simulink model "c00009M_harness"  (R2018a)
settings: Solver=FixedStepAuto  StartTime=0.0  StopTime=300  FixedStep=0.1  RelTol=1e-3
undefined symbols (not defined in the file): A1, hmax, PriorityTank, R1, R2, sigbuilder_block
(part 3 of 29)

== system c00009M_harness/Eval226 ==
  In1 : Inport
  In2 : Inport  Port=2
  Constant3 : Constant
  Data Type Conversion : DataTypeConversion
  Data Type Conversion1 : DataTypeConversion
  Memory1 : Memory  InitialCondition=1
  Memory2 : Memory  InitialCondition=1
  MinMax : MinMax  Inputs=3
  MinMax1 : MinMax  Inputs=2
  MinMax2 : MinMax  Inputs=2
  ROOut1 : RelationalOperator  Operator===  OutDataTypeStr=boolean  RndMeth=Simplest
  ROOut2 : RelationalOperator  Operator===  OutDataTypeStr=boolean  RndMeth=Simplest
  Out1 : Outport
  wires:
  Data Type Conversion1/1 -> MinMax2/1
  Data Type Conversion/1 -> MinMax1/1
  MinMax1/1 -> Memory1/1, MinMax/1
  MinMax2/1 -> MinMax/2, Memory2/1
  ROOut1/1 -> Data Type Conversion/1
  Memory2/1 -> MinMax2/2
  ROOut2/1 -> Data Type Conversion1/1
  Memory1/1 -> MinMax1/2
  [out2] -> ROOut2/2
  In1/1 -> ROOut1/1
  In2/1 -> ROOut2/1
  [out1] -> ROOut1/2
  MinMax/1 -> Out1/1
  Constant3/1 -> MinMax/3

== system c00009M_harness/Eval227 ==
  In1 : Inport
  In2 : Inport  Port=2
  Constant3 : Constant
  Data Type Conversion : DataTypeConversion
  Data Type Conversion1 : DataTypeConversion
  Memory1 : Memory  InitialCondition=1
  Memory2 : Memory  InitialCondition=1
  MinMax : MinMax  Inputs=3
  MinMax1 : MinMax  Inputs=2
  MinMax2 : MinMax  Inputs=2
  ROOut1 : RelationalOperator  Operator===  OutDataTypeStr=boolean  RndMeth=Simplest
  ROOut2 : RelationalOperator  Operator===  OutDataTypeStr=boolean  RndMeth=Simplest
  Out1 : Outport
  wires:
  Data Type Conversion1/1 -> MinMax2/1
  Data Type Conversion/1 -> MinMax1/1
  MinMax1/1 -> Memory1/1, MinMax/1
  MinMax2/1 -> MinMax/2, Memory2/1
  ROOut1/1 -> Data Type Conversion/1
  Memory2/1 -> MinMax2/2
  ROOut2/1 -> Data Type Conversion1/1
  Memory1/1 -> MinMax1/2
  [out2] -> ROOut2/2
  In1/1 -> ROOut1/1
  In2/1 -> ROOut2/1
  [out1] -> ROOut1/2
  MinMax/1 -> Out1/1
  Constant3/1 -> MinMax/3

== system c00009M_harness/Eval228 ==
  In1 : Inport
  In2 : Inport  Port=2
  Constant3 : Constant
  Data Type Conversion : DataTypeConversion
  Data Type Conversion1 : DataTypeConversion
  Memory1 : Memory  InitialCondition=1
  Memory2 : Memory  InitialCondition=1
  MinMax : MinMax  Inputs=3
  MinMax1 : MinMax  Inputs=2
  MinMax2 : MinMax  Inputs=2
  ROOut1 : RelationalOperator  Operator===  OutDataTypeStr=boolean  RndMeth=Simplest
  ROOut2 : RelationalOperator  Operator===  OutDataTypeStr=boolean  RndMeth=Simplest
  Out1 : Outport
  wires:
  Data Type Conversion1/1 -> MinMax2/1
  Data Type Conversion/1 -> MinMax1/1
  MinMax1/1 -> Memory1/1, MinMax/1
  MinMax2/1 -> MinMax/2, Memory2/1
  ROOut1/1 -> Data Type Conversion/1
  Memory2/1 -> MinMax2/2
  ROOut2/1 -> Data Type Conversion1/1
  Memory1/1 -> MinMax1/2
  [out2] -> ROOut2/2
  In1/1 -> ROOut1/1
  In2/1 -> ROOut2/1
  [out1] -> ROOut1/2
  MinMax/1 -> Out1/1
  Constant3/1 -> MinMax/3

== system c00009M_harness/Eval229 ==
  In1 : Inport
  In2 : Inport  Port=2
  Constant3 : Constant
  Data Type Conversion : DataTypeConversion
  Data Type Conversion1 : DataTypeConversion
  Memory1 : Memory  InitialCondition=1
  Memory2 : Memory  InitialCondition=1
  MinMax : MinMax  Inputs=3
  MinMax1 : MinMax  Inputs=2
  MinMax2 : MinMax  Inputs=2
  ROOut1 : RelationalOperator  Operator===  OutDataTypeStr=boolean  RndMeth=Simplest
  ROOut2 : RelationalOperator  Operator===  OutDataTypeStr=boolean  RndMeth=Simplest
  Out1 : Outport
  wires:
  Data Type Conversion1/1 -> MinMax2/1
  Data Type Conversion/1 -> MinMax1/1
  MinMax1/1 -> Memory1/1, MinMax/1
  MinMax2/1 -> MinMax/2, Memory2/1
  ROOut1/1 -> Data Type Conversion/1
  Memory2/1 -> MinMax2/2
  ROOut2/1 -> Data Type Conversion1/1
  Memory1/1 -> MinMax1/2
  [out2] -> ROOut2/2
  In1/1 -> ROOut1/1
  In2/1 -> ROOut2/1
  [out1] -> ROOut1/2
  MinMax/1 -> Out1/1
  Constant3/1 -> MinMax/3

== system c00009M_harness/Eval45 ==
  In1 : Inport
  In2 : Inport  Port=2
  Constant3 : Constant
  Data Type Conversion : DataTypeConversion
  Data Type Conversion1 : DataTypeConversion
  Memory1 : Memory  InitialCondition=1
  Memory2 : Memory  InitialCondition=1
  MinMax : MinMax  Inputs=3
  MinMax1 : MinMax  Inputs=2
  MinMax2 : MinMax  Inputs=2
  ROOut1 : RelationalOperator  Operator===  OutDataTypeStr=boolean  RndMeth=Simplest
  ROOut2 : RelationalOperator  Operator===  OutDataTypeStr=boolean  RndMeth=Simplest
  Out1 : Outport
  wires:
  Data Type Conversion1/1 -> MinMax2/1
  Data Type Conversion/1 -> MinMax1/1
  MinMax1/1 -> Memory1/1, MinMax/1
  MinMax2/1 -> MinMax/2, Memory2/1
  ROOut1/1 -> Data Type Conversion/1
  Memory2/1 -> MinMax2/2
  ROOut2/1 -> Data Type Conversion1/1
  Memory1/1 -> MinMax1/2
  [out2] -> ROOut2/2
  In1/1 -> ROOut1/1
  In2/1 -> ROOut2/1
  [out1] -> ROOut1/2
  MinMax/1 -> Out1/1
  Constant3/1 -> MinMax/3

== system c00009M_harness/Eval46 ==
  In1 : Inport
  In2 : Inport  Port=2
  Constant3 : Constant
  Data Type Conversion : DataTypeConversion
  Data Type Conversion1 : DataTypeConversion
  Memory1 : Memory  InitialCondition=1
  Memory2 : Memory  InitialCondition=1
  MinMax : MinMax  Inputs=3
  MinMax1 : MinMax  Inputs=2
  MinMax2 : MinMax  Inputs=2
  ROOut1 : RelationalOperator  Operator===  OutDataTypeStr=boolean  RndMeth=Simplest
  ROOut2 : RelationalOperator  Operator===  OutDataTypeStr=boolean  RndMeth=Simplest
  Out1 : Outport
  wires:
  Data Type Conversion1/1 -> MinMax2/1
  Data Type Conversion/1 -> MinMax1/1
  MinMax1/1 -> Memory1/1, MinMax/1
  MinMax2/1 -> MinMax/2, Memory2/1
  ROOut1/1 -> Data Type Conversion/1
  Memory2/1 -> MinMax2/2
  ROOut2/1 -> Data Type Conversion1/1
  Memory1/1 -> MinMax1/2
  [out2] -> ROOut2/2
  In1/1 -> ROOut1/1
  In2/1 -> ROOut2/1
  [out1] -> ROOut1/2
  MinMax/1 -> Out1/1
  Constant3/1 -> MinMax/3

== system c00009M_harness/Eval47 ==
  In1 : Inport
  In2 : Inport  Port=2
  Constant3 : Constant
  Data Type Conversion : DataTypeConversion
  Data Type Conversion1 : DataTypeConversion
  Memory1 : Memory  InitialCondition=1
  Memory2 : Memory  InitialCondition=1
  MinMax : MinMax  Inputs=3
  MinMax1 : MinMax  Inputs=2
  MinMax2 : MinMax  Inputs=2
  ROOut1 : RelationalOperator  Operator===  OutDataTypeStr=boolean  RndMeth=Simplest
  ROOut2 : RelationalOperator  Operator===  OutDataTypeStr=boolean  RndMeth=Simplest
  Out1 : Outport
  wires:
  Data Type Conversion1/1 -> MinMax2/1
  Data Type Conversion/1 -> MinMax1/1
  MinMax1/1 -> Memory1/1, MinMax/1
  MinMax2/1 -> MinMax/2, Memory2/1
  ROOut1/1 -> Data Type Conversion/1
  Memory2/1 -> MinMax2/2
  ROOut2/1 -> Data Type Conversion1/1
  Memory1/1 -> MinMax1/2
  [out2] -> ROOut2/2
  In1/1 -> ROOut1/1
  In2/1 -> ROOut2/1
  [out1] -> ROOut1/2
  MinMax/1 -> Out1/1
  Constant3/1 -> MinMax/3

== system c00009M_harness/Eval48 ==
  In1 : Inport
  In2 : Inport  Port=2
  Constant3 : Constant
  Data Type Conversion : DataTypeConversion
  Data Type Conversion1 : DataTypeConversion
  Memory1 : Memory  InitialCondition=1
  Memory2 : Memory  InitialCondition=1
  MinMax : MinMax  Inputs=3
  MinMax1 : MinMax  Inputs=2
  MinMax2 : MinMax  Inputs=2
  ROOut1 : RelationalOperator  Operator===  OutDataTypeStr=boolean  RndMeth=Simplest
  ROOut2 : RelationalOperator  Operator===  OutDataTypeStr=boolean  RndMeth=Simplest
  Out1 : Outport
  wires:
  Data Type Conversion1/1 -> MinMax2/1
  Data Type Conversion/1 -> MinMax1/1
  MinMax1/1 -> Memory1/1, MinMax/1
  MinMax2/1 -> MinMax/2, Memory2/1
  ROOut1/1 -> Data Type Conversion/1
  Memory2/1 -> MinMax2/2
  ROOut2/1 -> Data Type Conversion1/1
  Memory1/1 -> MinMax1/2
  [out2] -> ROOut2/2
  In1/1 -> ROOut1/1
  In2/1 -> ROOut2/1
  [out1] -> ROOut1/2
  MinMax/1 -> Out1/1
  Constant3/1 -> MinMax/3

== system c00009M_harness/Eval49 ==
  In1 : Inport
  In2 : Inport  Port=2
  Constant3 : Constant
  Data Type Conversion : DataTypeConversion
  Data Type Conversion1 : DataTypeConversion
  Memory1 : Memory  InitialCondition=1
  Memory2 : Memory  InitialCondition=1
  MinMax : MinMax  Inputs=3
  MinMax1 : MinMax  Inputs=2
  MinMax2 : MinMax  Inputs=2
  ROOut1 : RelationalOperator  Operator===  OutDataTypeStr=boolean  RndMeth=Simplest
  ROOut2 : RelationalOperator  Operator===  OutDataTypeStr=boolean  RndMeth=Simplest
  Out1 : Outport
  wires:
  Data Type Conversion1/1 -> MinMax2/1
  Data Type Conversion/1 -> MinMax1/1
  MinMax1/1 -> Memory1/1, MinMax/1
  MinMax2/1 -> MinMax/2, Memory2/1
  ROOut1/1 -> Data Type Conversion/1
  Memory2/1 -> MinMax2/2
  ROOut2/1 -> Data Type Conversion1/1
  Memory1/1 -> MinMax1/2
  [out2] -> ROOut2/2
  In1/1 -> ROOut1/1
  In2/1 -> ROOut2/1
  [out1] -> ROOut1/2
  MinMax/1 -> Out1/1
  Constant3/1 -> MinMax/3

== system c00009M_harness/Eval50 ==
  In1 : Inport
  In2 : Inport  Port=2
  Constant3 : Constant
  Data Type Conversion : DataTypeConversion
  Data Type Conversion1 : DataTypeConversion
  Memory1 : Memory  InitialCondition=1
  Memory2 : Memory  InitialCondition=1
  MinMax : MinMax  Inputs=3
  MinMax1 : MinMax  Inputs=2
  MinMax2 : MinMax  Inputs=2
  ROOut1 : RelationalOperator  Operator===  OutDataTypeStr=boolean  RndMeth=Simplest
  ROOut2 : RelationalOperator  Operator===  OutDataTypeStr=boolean  RndMeth=Simplest
  Out1 : Outport
  wires:
  Data Type Conversion1/1 -> MinMax2/1
  Data Type Conversion/1 -> MinMax1/1
  MinMax1/1 -> Memory1/1, MinMax/1
  MinMax2/1 -> MinMax/2, Memory2/1
  ROOut1/1 -> Data Type Conversion/1
  Memory2/1 -> MinMax2/2
  ROOut2/1 -> Data Type Conversion1/1
  Memory1/1 -> MinMax1/2
  [out2] -> ROOut2/2
  In1/1 -> ROOut1/1
  In2/1 -> ROOut2/1
  [out1] -> ROOut1/2
  MinMax/1 -> Out1/1
  Constant3/1 -> MinMax/3

== system c00009M_harness/Eval51 ==
  In1 : Inport
  In2 : Inport  Port=2
  Constant3 : Constant
  Data Type Conversion : DataTypeConversion
  Data Type Conversion1 : DataTypeConversion
  Memory1 : Memory  InitialCondition=1
  Memory2 : Memory  InitialCondition=1
  MinMax : MinMax  Inputs=3
  MinMax1 : MinMax  Inputs=2
  MinMax2 : MinMax  Inputs=2
  ROOut1 : RelationalOperator  Operator===  OutDataTypeStr=boolean  RndMeth=Simplest
  ROOut2 : RelationalOperator  Operator===  OutDataTypeStr=boolean  RndMeth=Simplest
  Out1 : Outport
  wires:
  Data Type Conversion1/1 -> MinMax2/1
  Data Type Conversion/1 -> MinMax1/1
  MinMax1/1 -> Memory1/1, MinMax/1
  MinMax2/1 -> MinMax/2, Memory2/1
  ROOut1/1 -> Data Type Conversion/1
  Memory2/1 -> MinMax2/2
  ROOut2/1 -> Data Type Conversion1/1
  Memory1/1 -> MinMax1/2
  [out2] -> ROOut2/2
  In1/1 -> ROOut1/1
  In2/1 -> ROOut2/1
  [out1] -> ROOut1/2
  MinMax/1 -> Out1/1
  Constant3/1 -> MinMax/3

== system c00009M_harness/Eval52 ==
  In1 : Inport
  In2 : Inport  Port=2
  Constant3 : Constant
  Data Type Conversion : DataTypeConversion
  Data Type Conversion1 : DataTypeConversion
  Memory1 : Memory  InitialCondition=1
  Memory2 : Memory  InitialCondition=1
  MinMax : MinMax  Inputs=3
  MinMax1 : MinMax  Inputs=2
  MinMax2 : MinMax  Inputs=2
  ROOut1 : RelationalOperator  Operator===  OutDataTypeStr=boolean  RndMeth=Simplest
  ROOut2 : RelationalOperator  Operator===  OutDataTypeStr=boolean  RndMeth=Simplest
  Out1 : Outport
  wires:
  Data Type Conversion1/1 -> MinMax2/1
  Data Type Conversion/1 -> MinMax1/1
  MinMax1/1 -> Memory1/1, MinMax/1
  MinMax2/1 -> MinMax/2, Memory2/1
  ROOut1/1 -> Data Type Conversion/1
  Memory2/1 -> MinMax2/2
  ROOut2/1 -> Data Type Conversion1/1
  Memory1/1 -> MinMax1/2
  [out2] -> ROOut2/2
  In1/1 -> ROOut1/1
  In2/1 -> ROOut2/1
  [out1] -> ROOut1/2
  MinMax/1 -> Out1/1
  Constant3/1 -> MinMax/3

== system c00009M_harness/Eval53 ==
  In1 : Inport
  In2 : Inport  Port=2
  Constant3 : Constant
  Data Type Conversion : DataTypeConversion
  Data Type Conversion1 : DataTypeConversion
  Memory1 : Memory  InitialCondition=1
  Memory2 : Memory  InitialCondition=1
  MinMax : MinMax  Inputs=3
  MinMax1 : MinMax  Inputs=2
  MinMax2 : MinMax  Inputs=2
  ROOut1 : RelationalOperator  Operator===  OutDataTypeStr=boolean  RndMeth=Simplest
  ROOut2 : RelationalOperator  Operator===  OutDataTypeStr=boolean  RndMeth=Simplest
  Out1 : Outport
  wires:
  Data Type Conversion1/1 -> MinMax2/1
  Data Type Conversion/1 -> MinMax1/1
  MinMax1/1 -> Memory1/1, MinMax/1
  MinMax2/1 -> MinMax/2, Memory2/1
  ROOut1/1 -> Data Type Conversion/1
  Memory2/1 -> MinMax2/2
  ROOut2/1 -> Data Type Conversion1/1
  Memory1/1 -> MinMax1/2
  [out2] -> ROOut2/2
  In1/1 -> ROOut1/1
  In2/1 -> ROOut2/1
  [out1] -> ROOut1/2
  MinMax/1 -> Out1/1
  Constant3/1 -> MinMax/3

== system c00009M_harness/Eval54 ==
  In1 : Inport
  In2 : Inport  Port=2
  Constant3 : Constant
  Data Type Conversion : DataTypeConversion
  Data Type Conversion1 : DataTypeConversion
  Memory1 : Memory  InitialCondition=1
  Memory2 : Memory  InitialCondition=1
  MinMax : MinMax  Inputs=3
  MinMax1 : MinMax  Inputs=2
  MinMax2 : MinMax  Inputs=2
  ROOut1 : RelationalOperator  Operator===  OutDataTypeStr=boolean  RndMeth=Simplest
  ROOut2 : RelationalOperator  Operator===  OutDataTypeStr=boolean  RndMeth=Simplest
  Out1 : Outport
  wires:
  Data Type Conversion1/1 -> MinMax2/1
  Data Type Conversion/1 -> MinMax1/1
  MinMax1/1 -> Memory1/1, MinMax/1
  MinMax2/1 -> MinMax/2, Memory2/1
  ROOut1/1 -> Data Type Conversion/1
  Memory2/1 -> MinMax2/2
  ROOut2/1 -> Data Type Conversion1/1
  Memory1/1 -> MinMax1/2
  [out2] -> ROOut2/2
  In1/1 -> ROOut1/1
  In2/1 -> ROOut2/1
  [out1] -> ROOut1/2
  MinMax/1 -> Out1/1
  Constant3/1 -> MinMax/3

== system c00009M_harness/Eval55 ==
  In1 : Inport
  In2 : Inport  Port=2
  Constant3 : Constant
  Data Type Conversion : DataTypeConversion
  Data Type Conversion1 : DataTypeConversion
  Memory1 : Memory  InitialCondition=1
  Memory2 : Memory  InitialCondition=1
  MinMax : MinMax  Inputs=3
  MinMax1 : MinMax  Inputs=2
  MinMax2 : MinMax  Inputs=2
  ROOut1 : RelationalOperator  Operator===  OutDataTypeStr=boolean  RndMeth=Simplest
  ROOut2 : RelationalOperator  Operator===  OutDataTypeStr=boolean  RndMeth=Simplest
  Out1 : Outport
  wires:
  Data Type Conversion1/1 -> MinMax2/1
  Data Type Conversion/1 -> MinMax1/1
  MinMax1/1 -> Memory1/1, MinMax/1
  MinMax2/1 -> MinMax/2, Memory2/1
  ROOut1/1 -> Data Type Conversion/1
  Memory2/1 -> MinMax2/2
  ROOut2/1 -> Data Type Conversion1/1
  Memory1/1 -> MinMax1/2
  [out2] -> ROOut2/2
  In1/1 -> ROOut1/1
  In2/1 -> ROOut2/1
  [out1] -> ROOut1/2
  MinMax/1 -> Out1/1
  Constant3/1 -> MinMax/3

== system c00009M_harness/Eval57 ==
  In1 : Inport
  In2 : Inport  Port=2
  Constant3 : Constant
  Data Type Conversion : DataTypeConversion
  Data Type Conversion1 : DataTypeConversion
  Memory1 : Memory  InitialCondition=1
  Memory2 : Memory  InitialCondition=1
  MinMax : MinMax  Inputs=3
  MinMax1 : MinMax  Inputs=2
  MinMax2 : MinMax  Inputs=2
  ROOut1 : RelationalOperator  Operator===  OutDataTypeStr=boolean  RndMeth=Simplest
  ROOut2 : RelationalOperator  Operator===  OutDataTypeStr=boolean  RndMeth=Simplest
  Out1 : Outport
  wires:
  Data Type Conversion1/1 -> MinMax2/1
  Data Type Conversion/1 -> MinMax1/1
  MinMax1/1 -> Memory1/1, MinMax/1
  MinMax2/1 -> MinMax/2, Memory2/1
  ROOut1/1 -> Data Type Conversion/1
  Memory2/1 -> MinMax2/2
  ROOut2/1 -> Data Type Conversion1/1
  Memory1/1 -> MinMax1/2
  [out2] -> ROOut2/2
  In1/1 -> ROOut1/1
  In2/1 -> ROOut2/1
  [out1] -> ROOut1/2
  MinMax/1 -> Out1/1
  Constant3/1 -> MinMax/3

== system c00009M_harness/Eval58 ==
  In1 : Inport
  In2 : Inport  Port=2
  Constant3 : Constant
  Data Type Conversion : DataTypeConversion
  Data Type Conversion1 : DataTypeConversion
  Memory1 : Memory  InitialCondition=1
  Memory2 : Memory  InitialCondition=1
  MinMax : MinMax  Inputs=3
  MinMax1 : MinMax  Inputs=2
  MinMax2 : MinMax  Inputs=2
  ROOut1 : RelationalOperator  Operator===  OutDataTypeStr=boolean  RndMeth=Simplest
  ROOut2 : RelationalOperator  Operator===  OutDataTypeStr=boolean  RndMeth=Simplest
  Out1 : Outport
  wires:
  Data Type Conversion1/1 -> MinMax2/1
  Data Type Conversion/1 -> MinMax1/1
  MinMax1/1 -> Memory1/1, MinMax/1
  MinMax2/1 -> MinMax/2, Memory2/1
  ROOut1/1 -> Data Type Conversion/1
  Memory2/1 -> MinMax2/2
  ROOut2/1 -> Data Type Conversion1/1
  Memory1/1 -> MinMax1/2
  [out2] -> ROOut2/2
  In1/1 -> ROOut1/1
  In2/1 -> ROOut2/1
  [out1] -> ROOut1/2
  MinMax/1 -> Out1/1
  Constant3/1 -> MinMax/3

== system c00009M_harness/Eval59 ==
  In1 : Inport
  In2 : Inport  Port=2
  Constant3 : Constant
  Data Type Conversion : DataTypeConversion
  Data Type Conversion1 : DataTypeConversion
  Memory1 : Memory  InitialCondition=1
  Memory2 : Memory  InitialCondition=1
  MinMax : MinMax  Inputs=3
  MinMax1 : MinMax  Inputs=2
  MinMax2 : MinMax  Inputs=2
  ROOut1 : RelationalOperator  Operator===  OutDataTypeStr=boolean  RndMeth=Simplest
  ROOut2 : RelationalOperator  Operator===  OutDataTypeStr=boolean  RndMeth=Simplest
  Out1 : Outport
  wires:
  Data Type Conversion1/1 -> MinMax2/1
  Data Type Conversion/1 -> MinMax1/1
  MinMax1/1 -> Memory1/1, MinMax/1
  MinMax2/1 -> MinMax/2, Memory2/1
  ROOut1/1 -> Data Type Conversion/1
  Memory2/1 -> MinMax2/2
  ROOut2/1 -> Data Type Conversion1/1
  Memory1/1 -> MinMax1/2
  [out2] -> ROOut2/2
  In1/1 -> ROOut1/1
  In2/1 -> ROOut2/1
  [out1] -> ROOut1/2
  MinMax/1 -> Out1/1
  Constant3/1 -> MinMax/3

== system c00009M_harness/Eval60 ==
  In1 : Inport
  In2 : Inport  Port=2
  Constant3 : Constant
  Data Type Conversion : DataTypeConversion
  Data Type Conversion1 : DataTypeConversion
  Memory1 : Memory  InitialCondition=1
  Memory2 : Memory  InitialCondition=1
  MinMax : MinMax  Inputs=3
  MinMax1 : MinMax  Inputs=2
  MinMax2 : MinMax  Inputs=2
  ROOut1 : RelationalOperator  Operator===  OutDataTypeStr=boolean  RndMeth=Simplest
  ROOut2 : RelationalOperator  Operator===  OutDataTypeStr=boolean  RndMeth=Simplest
  Out1 : Outport
  wires:
  Data Type Conversion1/1 -> MinMax2/1
  Data Type Conversion/1 -> MinMax1/1
  MinMax1/1 -> Memory1/1, MinMax/1
  MinMax2/1 -> MinMax/2, Memory2/1
  ROOut1/1 -> Data Type Conversion/1
  Memory2/1 -> MinMax2/2
  ROOut2/1 -> Data Type Conversion1/1
  Memory1/1 -> MinMax1/2
  [out2] -> ROOut2/2
  In1/1 -> ROOut1/1
  In2/1 -> ROOut2/1
  [out1] -> ROOut1/2
  MinMax/1 -> Out1/1
  Constant3/1 -> MinMax/3

== system c00009M_harness/Eval61 ==
  In1 : Inport
  In2 : Inport  Port=2
  Constant3 : Constant
  Data Type Conversion : DataTypeConversion
  Data Type Conversion1 : DataTypeConversion
  Memory1 : Memory  InitialCondition=1
  Memory2 : Memory  InitialCondition=1
  MinMax : MinMax  Inputs=3
  MinMax1 : MinMax  Inputs=2
  MinMax2 : MinMax  Inputs=2
  ROOut1 : RelationalOperator  Operator===  OutDataTypeStr=boolean  RndMeth=Simplest
  ROOut2 : RelationalOperator  Operator===  OutDataTypeStr=boolean  RndMeth=Simplest
  Out1 : Outport
  wires:
  Data Type Conversion1/1 -> MinMax2/1
  Data Type Conversion/1 -> MinMax1/1
  MinMax1/1 -> Memory1/1, MinMax/1
  MinMax2/1 -> MinMax/2, Memory2/1
  ROOut1/1 -> Data Type Conversion/1
  Memory2/1 -> MinMax2/2
  ROOut2/1 -> Data Type Conversion1/1
  Memory1/1 -> MinMax1/2
  [out2] -> ROOut2/2
  In1/1 -> ROOut1/1
  In2/1 -> ROOut2/1
  [out1] -> ROOut1/2
  MinMax/1 -> Out1/1
  Constant3/1 -> MinMax/3

== system c00009M_harness/Eval62 ==
  In1 : Inport
  In2 : Inport  Port=2
  Constant3 : Constant
  Data Type Conversion : DataTypeConversion
  Data Type Conversion1 : DataTypeConversion
  Memory1 : Memory  InitialCondition=1
  Memory2 : Memory  InitialCondition=1
  MinMax : MinMax  Inputs=3
  MinMax1 : MinMax  Inputs=2
  MinMax2 : MinMax  Inputs=2
  ROOut1 : RelationalOperator  Operator===  OutDataTypeStr=boolean  RndMeth=Simplest
  ROOut2 : RelationalOperator  Operator===  OutDataTypeStr=boolean  RndMeth=Simplest
  Out1 : Outport
  wires:
  Data Type Conversion1/1 -> MinMax2/1
  Data Type Conversion/1 -> MinMax1/1
  MinMax1/1 -> Memory1/1, MinMax/1
  MinMax2/1 -> MinMax/2, Memory2/1
  ROOut1/1 -> Data Type Conversion/1
  Memory2/1 -> MinMax2/2
  ROOut2/1 -> Data Type Conversion1/1
  Memory1/1 -> MinMax1/2
  [out2] -> ROOut2/2
  In1/1 -> ROOut1/1
  In2/1 -> ROOut2/1
  [out1] -> ROOut1/2
  MinMax/1 -> Out1/1
  Constant3/1 -> MinMax/3

== system c00009M_harness/Eval63 ==
  In1 : Inport
  In2 : Inport  Port=2
  Constant3 : Constant
  Data Type Conversion : DataTypeConversion
  Data Type Conversion1 : DataTypeConversion
  Memory1 : Memory  InitialCondition=1
  Memory2 : Memory  InitialCondition=1
  MinMax : MinMax  Inputs=3
  MinMax1 : MinMax  Inputs=2
  MinMax2 : MinMax  Inputs=2
  ROOut1 : RelationalOperator  Operator===  OutDataTypeStr=boolean  RndMeth=Simplest
  ROOut2 : RelationalOperator  Operator===  OutDataTypeStr=boolean  RndMeth=Simplest
  Out1 : Outport
  wires:
  Data Type Conversion1/1 -> MinMax2/1
  Data Type Conversion/1 -> MinMax1/1
  MinMax1/1 -> Memory1/1, MinMax/1
  MinMax2/1 -> MinMax/2, Memory2/1
  ROOut1/1 -> Data Type Conversion/1
  Memory2/1 -> MinMax2/2
  ROOut2/1 -> Data Type Conversion1/1
  Memory1/1 -> MinMax1/2
  [out2] -> ROOut2/2
  In1/1 -> ROOut1/1
  In2/1 -> ROOut2/1
  [out1] -> ROOut1/2
  MinMax/1 -> Out1/1
  Constant3/1 -> MinMax/3

== system c00009M_harness/Eval64 ==
  In1 : Inport
  In2 : Inport  Port=2
  Constant3 : Constant
  Data Type Conversion : DataTypeConversion
  Data Type Conversion1 : DataTypeConversion
  Memory1 : Memory  InitialCondition=1
  Memory2 : Memory  InitialCondition=1
  MinMax : MinMax  Inputs=3
  MinMax1 : MinMax  Inputs=2
  MinMax2 : MinMax  Inputs=2
  ROOut1 : RelationalOperator  Operator===  OutDataTypeStr=boolean  RndMeth=Simplest
  ROOut2 : RelationalOperator  Operator===  OutDataTypeStr=boolean  RndMeth=Simplest
  Out1 : Outport
  wires:
  Data Type Conversion1/1 -> MinMax2/1
  Data Type Conversion/1 -> MinMax1/1
  MinMax1/1 -> Memory1/1, MinMax/1
  MinMax2/1 -> MinMax/2, Memory2/1
  ROOut1/1 -> Data Type Conversion/1
  Memory2/1 -> MinMax2/2
  ROOut2/1 -> Data Type Conversion1/1
  Memory1/1 -> MinMax1/2
  [out2] -> ROOut2/2
  In1/1 -> ROOut1/1
  In2/1 -> ROOut2/1
  [out1] -> ROOut1/2
  MinMax/1 -> Out1/1
  Constant3/1 -> MinMax/3

== system c00009M_harness/Eval65 ==
  In1 : Inport
  In2 : Inport  Port=2
  Constant3 : Constant
  Data Type Conversion : DataTypeConversion
  Data Type Conversion1 : DataTypeConversion
  Memory1 : Memory  InitialCondition=1
  Memory2 : Memory  InitialCondition=1
  MinMax : MinMax  Inputs=3
  MinMax1 : MinMax  Inputs=2
  MinMax2 : MinMax  Inputs=2
  ROOut1 : RelationalOperator  Operator===  OutDataTypeStr=boolean  RndMeth=Simplest
  ROOut2 : RelationalOperator  Operator===  OutDataTypeStr=boolean  RndMeth=Simplest
  Out1 : Outport
  wires:
  Data Type Conversion1/1 -> MinMax2/1
  Data Type Conversion/1 -> MinMax1/1
  MinMax1/1 -> Memory1/1, MinMax/1
  MinMax2/1 -> MinMax/2, Memory2/1
  ROOut1/1 -> Data Type Conversion/1
  Memory2/1 -> MinMax2/2
  ROOut2/1 -> Data Type Conversion1/1
  Memory1/1 -> MinMax1/2
  [out2] -> ROOut2/2
  In1/1 -> ROOut1/1
  In2/1 -> ROOut2/1
  [out1] -> ROOut1/2
  MinMax/1 -> Out1/1
  Constant3/1 -> MinMax/3

== system c00009M_harness/Eval66 ==
  In1 : Inport
  In2 : Inport  Port=2
  Constant3 : Constant
  Data Type Conversion : DataTypeConversion
  Data Type Conversion1 : DataTypeConversion
  Memory1 : Memory  InitialCondition=1
  Memory2 : Memory  InitialCondition=1
  MinMax : MinMax  Inputs=3
  MinMax1 : MinMax  Inputs=2
  MinMax2 : MinMax  Inputs=2
  ROOut1 : RelationalOperator  Operator===  OutDataTypeStr=boolean  RndMeth=Simplest
  ROOut2 : RelationalOperator  Operator===  OutDataTypeStr=boolean  RndMeth=Simplest
  Out1 : Outport
  wires:
  Data Type Conversion1/1 -> MinMax2/1
  Data Type Conversion/1 -> MinMax1/1
  MinMax1/1 -> Memory1/1, MinMax/1
  MinMax2/1 -> MinMax/2, Memory2/1
  ROOut1/1 -> Data Type Conversion/1
  Memory2/1 -> MinMax2/2
  ROOut2/1 -> Data Type Conversion1/1
  Memory1/1 -> MinMax1/2
  [out2] -> ROOut2/2
  In1/1 -> ROOut1/1
  In2/1 -> ROOut2/1
  [out1] -> ROOut1/2
  MinMax/1 -> Out1/1
  Constant3/1 -> MinMax/3

== system c00009M_harness/Eval67 ==
  In1 : Inport
  In2 : Inport  Port=2
  Constant3 : Constant
  Data Type Conversion : DataTypeConversion
  Data Type Conversion1 : DataTypeConversion
  Memory1 : Memory  InitialCondition=1
  Memory2 : Memory  InitialCondition=1
  MinMax : MinMax  Inputs=3
  MinMax1 : MinMax  Inputs=2
  MinMax2 : MinMax  Inputs=2
  ROOut1 : RelationalOperator  Operator===  OutDataTypeStr=boolean  RndMeth=Simplest
  ROOut2 : RelationalOperator  Operator===  OutDataTypeStr=boolean  RndMeth=Simplest
  Out1 : Outport
  wires:
  Data Type Conversion1/1 -> MinMax2/1
  Data Type Conversion/1 -> MinMax1/1
  MinMax1/1 -> Memory1/1, MinMax/1
  MinMax2/1 -> MinMax/2, Memory2/1
  ROOut1/1 -> Data Type Conversion/1
  Memory2/1 -> MinMax2/2
  ROOut2/1 -> Data Type Conversion1/1
  Memory1/1 -> MinMax1/2
  [out2] -> ROOut2/2
  In1/1 -> ROOut1/1
  In2/1 -> ROOut2/1
  [out1] -> ROOut1/2
  MinMax/1 -> Out1/1
  Constant3/1 -> MinMax/3

== system c00009M_harness/Eval68 ==
  In1 : Inport
  In2 : Inport  Port=2
  Constant3 : Constant
  Data Type Conversion : DataTypeConversion
  Data Type Conversion1 : DataTypeConversion
  Memory1 : Memory  InitialCondition=1
  Memory2 : Memory  InitialCondition=1
  MinMax : MinMax  Inputs=3
  MinMax1 : MinMax  Inputs=2
  MinMax2 : MinMax  Inputs=2
  ROOut1 : RelationalOperator  Operator===  OutDataTypeStr=boolean  RndMeth=Simplest
  ROOut2 : RelationalOperator  Operator===  OutDataTypeStr=boolean  RndMeth=Simplest
  Out1 : Outport
  wires:
  Data Type Conversion1/1 -> MinMax2/1
  Data Type Conversion/1 -> MinMax1/1
  MinMax1/1 -> Memory1/1, MinMax/1
  MinMax2/1 -> MinMax/2, Memory2/1
  ROOut1/1 -> Data Type Conversion/1
  Memory2/1 -> MinMax2/2
  ROOut2/1 -> Data Type Conversion1/1
  Memory1/1 -> MinMax1/2
  [out2] -> ROOut2/2
  In1/1 -> ROOut1/1
  In2/1 -> ROOut2/1
  [out1] -> ROOut1/2
  MinMax/1 -> Out1/1
  Constant3/1 -> MinMax/3

== system c00009M_harness/Eval69 ==
  In1 : Inport
  In2 : Inport  Port=2
  Constant3 : Constant
  Data Type Conversion : DataTypeConversion
  Data Type Conversion1 : DataTypeConversion
  Memory1 : Memory  InitialCondition=1
  Memory2 : Memory  InitialCondition=1
  MinMax : MinMax  Inputs=3
  MinMax1 : MinMax  Inputs=2
  MinMax2 : MinMax  Inputs=2
  ROOut1 : RelationalOperator  Operator===  OutDataTypeStr=boolean  RndMeth=Simplest
  ROOut2 : RelationalOperator  Operator===  OutDataTypeStr=boolean  RndMeth=Simplest
  Out1 : Outport
  wires:
  Data Type Conversion1/1 -> MinMax2/1
  Data Type Conversion/1 -> MinMax1/1
  MinMax1/1 -> Memory1/1, MinMax/1
  MinMax2/1 -> MinMax/2, Memory2/1
  ROOut1/1 -> Data Type Conversion/1
  Memory2/1 -> MinMax2/2
  ROOut2/1 -> Data Type Conversion1/1
  Memory1/1 -> MinMax1/2
  [out2] -> ROOut2/2
  In1/1 -> ROOut1/1
  In2/1 -> ROOut2/1
  [out1] -> ROOut1/2
  MinMax/1 -> Out1/1
  Constant3/1 -> MinMax/3

== system c00009M_harness/Eval70 ==
  In1 : Inport
  In2 : Inport  Port=2
  Constant3 : Constant
  Data Type Conversion : DataTypeConversion
  Data Type Conversion1 : DataTypeConversion
  Memory1 : Memory  InitialCondition=1
  Memory2 : Memory  InitialCondition=1
  MinMax : MinMax  Inputs=3
  MinMax1 : MinMax  Inputs=2
  MinMax2 : MinMax  Inputs=2
  ROOut1 : RelationalOperator  Operator===  OutDataTypeStr=boolean  RndMeth=Simplest
  ROOut2 : RelationalOperator  Operator===  OutDataTypeStr=boolean  RndMeth=Simplest
  Out1 : Outport
  wires:
  Data Type Conversion1/1 -> MinMax2/1
  Data Type Conversion/1 -> MinMax1/1
  MinMax1/1 -> Memory1/1, MinMax/1
  MinMax2/1 -> MinMax/2, Memory2/1
  ROOut1/1 -> Data Type Conversion/1
  Memory2/1 -> MinMax2/2
  ROOut2/1 -> Data Type Conversion1/1
  Memory1/1 -> MinMax1/2
  [out2] -> ROOut2/2
  In1/1 -> ROOut1/1
  In2/1 -> ROOut2/1
  [out1] -> ROOut1/2
  MinMax/1 -> Out1/1
  Constant3/1 -> MinMax/3

== system c00009M_harness/Eval71 ==
  In1 : Inport
  In2 : Inport  Port=2
  Constant3 : Constant
  Data Type Conversion : DataTypeConversion
  Data Type Conversion1 : DataTypeConversion
  Memory1 : Memory  InitialCondition=1
  Memory2 : Memory  InitialCondition=1
  MinMax : MinMax  Inputs=3
  MinMax1 : MinMax  Inputs=2
  MinMax2 : MinMax  Inputs=2
  ROOut1 : RelationalOperator  Operator===  OutDataTypeStr=boolean  RndMeth=Simplest
  ROOut2 : RelationalOperator  Operator===  OutDataTypeStr=boolean  RndMeth=Simplest
  Out1 : Outport
  wires:
  Data Type Conversion1/1 -> MinMax2/1
  Data Type Conversion/1 -> MinMax1/1
  MinMax1/1 -> Memory1/1, MinMax/1
  MinMax2/1 -> MinMax/2, Memory2/1
  ROOut1/1 -> Data Type Conversion/1
  Memory2/1 -> MinMax2/2
  ROOut2/1 -> Data Type Conversion1/1
  Memory1/1 -> MinMax1/2
  [out2] -> ROOut2/2
  In1/1 -> ROOut1/1
  In2/1 -> ROOut2/1
  [out1] -> ROOut1/2
  MinMax/1 -> Out1/1
  Constant3/1 -> MinMax/3

== system c00009M_harness/Eval72 ==
  In1 : Inport
  In2 : Inport  Port=2
  Constant3 : Constant
  Data Type Conversion : DataTypeConversion
  Data Type Conversion1 : DataTypeConversion
  Memory1 : Memory  InitialCondition=1
  Memory2 : Memory  InitialCondition=1
  MinMax : MinMax  Inputs=3
  MinMax1 : MinMax  Inputs=2
  MinMax2 : MinMax  Inputs=2
  ROOut1 : RelationalOperator  Operator===  OutDataTypeStr=boolean  RndMeth=Simplest
  ROOut2 : RelationalOperator  Operator===  OutDataTypeStr=boolean  RndMeth=Simplest
  Out1 : Outport
  wires:
  Data Type Conversion1/1 -> MinMax2/1
  Data Type Conversion/1 -> MinMax1/1
  MinMax1/1 -> Memory1/1, MinMax/1
  MinMax2/1 -> MinMax/2, Memory2/1
  ROOut1/1 -> Data Type Conversion/1
  Memory2/1 -> MinMax2/2
  ROOut2/1 -> Data Type Conversion1/1
  Memory1/1 -> MinMax1/2
  [out2] -> ROOut2/2
  In1/1 -> ROOut1/1
  In2/1 -> ROOut2/1
  [out1] -> ROOut1/2
  MinMax/1 -> Out1/1
  Constant3/1 -> MinMax/3

== system c00009M_harness/Eval73 ==
  In1 : Inport
  In2 : Inport  Port=2
  Constant3 : Constant
  Data Type Conversion : DataTypeConversion
  Data Type Conversion1 : DataTypeConversion
  Memory1 : Memory  InitialCondition=1
  Memory2 : Memory  InitialCondition=1
  MinMax : MinMax  Inputs=3
  MinMax1 : MinMax  Inputs=2
  MinMax2 : MinMax  Inputs=2
  ROOut1 : RelationalOperator  Operator===  OutDataTypeStr=boolean  RndMeth=Simplest
  ROOut2 : RelationalOperator  Operator===  OutDataTypeStr=boolean  RndMeth=Simplest
  Out1 : Outport
  wires:
  Data Type Conversion1/1 -> MinMax2/1
  Data Type Conversion/1 -> MinMax1/1
  MinMax1/1 -> Memory1/1, MinMax/1
  MinMax2/1 -> MinMax/2, Memory2/1
  ROOut1/1 -> Data Type Conversion/1
  Memory2/1 -> MinMax2/2
  ROOut2/1 -> Data Type Conversion1/1
  Memory1/1 -> MinMax1/2
  [out2] -> ROOut2/2
  In1/1 -> ROOut1/1
  In2/1 -> ROOut2/1
  [out1] -> ROOut1/2
  MinMax/1 -> Out1/1
  Constant3/1 -> MinMax/3

== system c00009M_harness/Eval74 ==
  In1 : Inport
  In2 : Inport  Port=2
  Constant3 : Constant
  Data Type Conversion : DataTypeConversion
  Data Type Conversion1 : DataTypeConversion
  Memory1 : Memory  InitialCondition=1
  Memory2 : Memory  InitialCondition=1
  MinMax : MinMax  Inputs=3
  MinMax1 : MinMax  Inputs=2
  MinMax2 : MinMax  Inputs=2
  ROOut1 : RelationalOperator  Operator===  OutDataTypeStr=boolean  RndMeth=Simplest
  ROOut2 : RelationalOperator  Operator===  OutDataTypeStr=boolean  RndMeth=Simplest
  Out1 : Outport
  wires:
  Data Type Conversion1/1 -> MinMax2/1
  Data Type Conversion/1 -> MinMax1/1
  MinMax1/1 -> Memory1/1, MinMax/1
  MinMax2/1 -> MinMax/2, Memory2/1
  ROOut1/1 -> Data Type Conversion/1
  Memory2/1 -> MinMax2/2
  ROOut2/1 -> Data Type Conversion1/1
  Memory1/1 -> MinMax1/2
  [out2] -> ROOut2/2
  In1/1 -> ROOut1/1
  In2/1 -> ROOut2/1
  [out1] -> ROOut1/2
  MinMax/1 -> Out1/1
  Constant3/1 -> MinMax/3

== system c00009M_harness/Eval75 ==
  In1 : Inport
  In2 : Inport  Port=2
  Constant3 : Constant
  Data Type Conversion : DataTypeConversion
  Data Type Conversion1 : DataTypeConversion
  Memory1 : Memory  InitialCondition=1
  Memory2 : Memory  InitialCondition=1
  MinMax : MinMax  Inputs=3
  MinMax1 : MinMax  Inputs=2
  MinMax2 : MinMax  Inputs=2
  ROOut1 : RelationalOperator  Operator===  OutDataTypeStr=boolean  RndMeth=Simplest
  ROOut2 : RelationalOperator  Operator===  OutDataTypeStr=boolean  RndMeth=Simplest
  Out1 : Outport
  wires:
  Data Type Conversion1/1 -> MinMax2/1
  Data Type Conversion/1 -> MinMax1/1
  MinMax1/1 -> Memory1/1, MinMax/1
  MinMax2/1 -> MinMax/2, Memory2/1
  ROOut1/1 -> Data Type Conversion/1
  Memory2/1 -> MinMax2/2
  ROOut2/1 -> Data Type Conversion1/1
  Memory1/1 -> MinMax1/2
  [out2] -> ROOut2/2
  In1/1 -> ROOut1/1
  In2/1 -> ROOut2/1
  [out1] -> ROOut1/2
  MinMax/1 -> Out1/1
  Constant3/1 -> MinMax/3

== system c00009M_harness/Eval76 ==
  In1 : Inport
  In2 : Inport  Port=2
  Constant3 : Constant
  Data Type Conversion : DataTypeConversion
  Data Type Conversion1 : DataTypeConversion
  Memory1 : Memory  InitialCondition=1
  Memory2 : Memory  InitialCondition=1
  MinMax : MinMax  Inputs=3
  MinMax1 : MinMax  Inputs=2
  MinMax2 : MinMax  Inputs=2
  ROOut1 : RelationalOperator  Operator===  OutDataTypeStr=boolean  RndMeth=Simplest
  ROOut2 : RelationalOperator  Operator===  OutDataTypeStr=boolean  RndMeth=Simplest
  Out1 : Outport
  wires:
  Data Type Conversion1/1 -> MinMax2/1
  Data Type Conversion/1 -> MinMax1/1
  MinMax1/1 -> Memory1/1, MinMax/1
  MinMax2/1 -> MinMax/2, Memory2/1
  ROOut1/1 -> Data Type Conversion/1
  Memory2/1 -> MinMax2/2
  ROOut2/1 -> Data Type Conversion1/1
  Memory1/1 -> MinMax1/2
  [out2] -> ROOut2/2
  In1/1 -> ROOut1/1
  In2/1 -> ROOut2/1
  [out1] -> ROOut1/2
  MinMax/1 -> Out1/1
  Constant3/1 -> MinMax/3

== system c00009M_harness/Eval77 ==
  In1 : Inport
  In2 : Inport  Port=2
  Constant3 : Constant
  Data Type Conversion : DataTypeConversion
  Data Type Conversion1 : DataTypeConversion
  Memory1 : Memory  InitialCondition=1
  Memory2 : Memory  InitialCondition=1
  MinMax : MinMax  Inputs=3
  MinMax1 : MinMax  Inputs=2
  MinMax2 : MinMax  Inputs=2
  ROOut1 : RelationalOperator  Operator===  OutDataTypeStr=boolean  RndMeth=Simplest
  ROOut2 : RelationalOperator  Operator===  OutDataTypeStr=boolean  RndMeth=Simplest
  Out1 : Outport
  wires:
  Data Type Conversion1/1 -> MinMax2/1
  Data Type Conversion/1 -> MinMax1/1
  MinMax1/1 -> Memory1/1, MinMax/1
  MinMax2/1 -> MinMax/2, Memory2/1
  ROOut1/1 -> Data Type Conversion/1
  Memory2/1 -> MinMax2/2
  ROOut2/1 -> Data Type Conversion1/1
  Memory1/1 -> MinMax1/2
  [out2] -> ROOut2/2
  In1/1 -> ROOut1/1
  In2/1 -> ROOut2/1
  [out1] -> ROOut1/2
  MinMax/1 -> Out1/1
  Constant3/1 -> MinMax/3

== system c00009M_harness/Eval78 ==
  In1 : Inport
  In2 : Inport  Port=2
  Constant3 : Constant
  Data Type Conversion : DataTypeConversion
  Data Type Conversion1 : DataTypeConversion
  Memory1 : Memory  InitialCondition=1
  Memory2 : Memory  InitialCondition=1
  MinMax : MinMax  Inputs=3
  MinMax1 : MinMax  Inputs=2
  MinMax2 : MinMax  Inputs=2
  ROOut1 : RelationalOperator  Operator===  OutDataTypeStr=boolean  RndMeth=Simplest
  ROOut2 : RelationalOperator  Operator===  OutDataTypeStr=boolean  RndMeth=Simplest
  Out1 : Outport
  wires:
  Data Type Conversion1/1 -> MinMax2/1
  Data Type Conversion/1 -> MinMax1/1
  MinMax1/1 -> Memory1/1, MinMax/1
  MinMax2/1 -> MinMax/2, Memory2/1
  ROOut1/1 -> Data Type Conversion/1
  Memory2/1 -> MinMax2/2
  ROOut2/1 -> Data Type Conversion1/1
  Memory1/1 -> MinMax1/2
  [out2] -> ROOut2/2
  In1/1 -> ROOut1/1
  In2/1 -> ROOut2/1
  [out1] -> ROOut1/2
  MinMax/1 -> Out1/1
  Constant3/1 -> MinMax/3

== system c00009M_harness/Eval79 ==
  In1 : Inport
  In2 : Inport  Port=2
  Constant3 : Constant
  Data Type Conversion : DataTypeConversion
  Data Type Conversion1 : DataTypeConversion
  Memory1 : Memory  InitialCondition=1
  Memory2 : Memory  InitialCondition=1
  MinMax : MinMax  Inputs=3
  MinMax1 : MinMax  Inputs=2
  MinMax2 : MinMax  Inputs=2
  ROOut1 : RelationalOperator  Operator===  OutDataTypeStr=boolean  RndMeth=Simplest
  ROOut2 : RelationalOperator  Operator===  OutDataTypeStr=boolean  RndMeth=Simplest
  Out1 : Outport
  wires:
  Data Type Conversion1/1 -> MinMax2/1
  Data Type Conversion/1 -> MinMax1/1
  MinMax1/1 -> Memory1/1, MinMax/1
  MinMax2/1 -> MinMax/2, Memory2/1
  ROOut1/1 -> Data Type Conversion/1
  Memory2/1 -> MinMax2/2
  ROOut2/1 -> Data Type Conversion1/1
  Memory1/1 -> MinMax1/2
  [out2] -> ROOut2/2
  In1/1 -> ROOut1/1
  In2/1 -> ROOut2/1
  [out1] -> ROOut1/2
  MinMax/1 -> Out1/1
  Constant3/1 -> MinMax/3

== system c00009M_harness/Eval80 ==
  In1 : Inport
  In2 : Inport  Port=2
  Constant3 : Constant
  Data Type Conversion : DataTypeConversion
  Data Type Conversion1 : DataTypeConversion
  Memory1 : Memory  InitialCondition=1
  Memory2 : Memory  InitialCondition=1
  MinMax : MinMax  Inputs=3
  MinMax1 : MinMax  Inputs=2
  MinMax2 : MinMax  Inputs=2
  ROOut1 : RelationalOperator  Operator===  OutDataTypeStr=boolean  RndMeth=Simplest
  ROOut2 : RelationalOperator  Operator===  OutDataTypeStr=boolean  RndMeth=Simplest
  Out1 : Outport
  wires:
  Data Type Conversion1/1 -> MinMax2/1
  Data Type Conversion/1 -> MinMax1/1
  MinMax1/1 -> Memory1/1, MinMax/1
  MinMax2/1 -> MinMax/2, Memory2/1
  ROOut1/1 -> Data Type Conversion/1
  Memory2/1 -> MinMax2/2
  ROOut2/1 -> Data Type Conversion1/1
  Memory1/1 -> MinMax1/2
  [out2] -> ROOut2/2
  In1/1 -> ROOut1/1
  In2/1 -> ROOut2/1
  [out1] -> ROOut1/2
  MinMax/1 -> Out1/1
  Constant3/1 -> MinMax/3

== system c00009M_harness/Eval81 ==
  In1 : Inport
  In2 : Inport  Port=2
  Constant3 : Constant
  Data Type Conversion : DataTypeConversion
  Data Type Conversion1 : DataTypeConversion
  Memory1 : Memory  InitialCondition=1
  Memory2 : Memory  InitialCondition=1
  MinMax : MinMax  Inputs=3
  MinMax1 : MinMax  Inputs=2
  MinMax2 : MinMax  Inputs=2
  ROOut1 : RelationalOperator  Operator===  OutDataTypeStr=boolean  RndMeth=Simplest
  ROOut2 : RelationalOperator  Operator===  OutDataTypeStr=boolean  RndMeth=Simplest
  Out1 : Outport
  wires:
  Data Type Conversion1/1 -> MinMax2/1
  Data Type Conversion/1 -> MinMax1/1
  MinMax1/1 -> Memory1/1, MinMax/1
  MinMax2/1 -> MinMax/2, Memory2/1
  ROOut1/1 -> Data Type Conversion/1
  Memory2/1 -> MinMax2/2
  ROOut2/1 -> Data Type Conversion1/1
  Memory1/1 -> MinMax1/2
  [out2] -> ROOut2/2
  In1/1 -> ROOut1/1
  In2/1 -> ROOut2/1
  [out1] -> ROOut1/2
  MinMax/1 -> Out1/1
  Constant3/1 -> MinMax/3

== system c00009M_harness/Eval82 ==
  In1 : Inport
  In2 : Inport  Port=2
  Constant3 : Constant
  Data Type Conversion : DataTypeConversion
  Data Type Conversion1 : DataTypeConversion
  Memory1 : Memory  InitialCondition=1
  Memory2 : Memory  InitialCondition=1
  MinMax : MinMax  Inputs=3
  MinMax1 : MinMax  Inputs=2
  MinMax2 : MinMax  Inputs=2
  ROOut1 : RelationalOperator  Operator===  OutDataTypeStr=boolean  RndMeth=Simplest
  ROOut2 : RelationalOperator  Operator===  OutDataTypeStr=boolean  RndMeth=Simplest
  Out1 : Outport
  wires:
  Data Type Conversion1/1 -> MinMax2/1
  Data Type Conversion/1 -> MinMax1/1
  MinMax1/1 -> Memory1/1, MinMax/1
  MinMax2/1 -> MinMax/2, Memory2/1
  ROOut1/1 -> Data Type Conversion/1
  Memory2/1 -> MinMax2/2
  ROOut2/1 -> Data Type Conversion1/1
  Memory1/1 -> MinMax1/2
  [out2] -> ROOut2/2
  In1/1 -> ROOut1/1
  In2/1 -> ROOut2/1
  [out1] -> ROOut1/2
  MinMax/1 -> Out1/1
  Constant3/1 -> MinMax/3

== system c00009M_harness/Eval86 ==
  In1 : Inport
  In2 : Inport  Port=2
  Constant3 : Constant
  Data Type Conversion : DataTypeConversion
  Data Type Conversion1 : DataTypeConversion
  Memory1 : Memory  InitialCondition=1
  Memory2 : Memory  InitialCondition=1
  MinMax : MinMax  Inputs=3
  MinMax1 : MinMax  Inputs=2
  MinMax2 : MinMax  Inputs=2
  ROOut1 : RelationalOperator  Operator===  OutDataTypeStr=boolean  RndMeth=Simplest
  ROOut2 : RelationalOperator  Operator===  OutDataTypeStr=boolean  RndMeth=Simplest
  Out1 : Outport
  wires:
  Data Type Conversion1/1 -> MinMax2/1
  Data Type Conversion/1 -> MinMax1/1
  MinMax1/1 -> Memory1/1, MinMax/1
  MinMax2/1 -> MinMax/2, Memory2/1
  ROOut1/1 -> Data Type Conversion/1
  Memory2/1 -> MinMax2/2
  ROOut2/1 -> Data Type Conversion1/1
  Memory1/1 -> MinMax1/2
  [out2] -> ROOut2/2
  In1/1 -> ROOut1/1
  In2/1 -> ROOut2/1
  [out1] -> ROOut1/2
  MinMax/1 -> Out1/1
  Constant3/1 -> MinMax/3

== system c00009M_harness/Eval87 ==
  In1 : Inport
  In2 : Inport  Port=2
  Constant3 : Constant
  Data Type Conversion : DataTypeConversion
  Data Type Conversion1 : DataTypeConversion
  Memory1 : Memory  InitialCondition=1
  Memory2 : Memory  InitialCondition=1
  MinMax : MinMax  Inputs=3
  MinMax1 : MinMax  Inputs=2
  MinMax2 : MinMax  Inputs=2
  ROOut1 : RelationalOperator  Operator===  OutDataTypeStr=boolean  RndMeth=Simplest
  ROOut2 : RelationalOperator  Operator===  OutDataTypeStr=boolean  RndMeth=Simplest
  Out1 : Outport
  wires:
  Data Type Conversion1/1 -> MinMax2/1
  Data Type Conversion/1 -> MinMax1/1
  MinMax1/1 -> Memory1/1, MinMax/1
  MinMax2/1 -> MinMax/2, Memory2/1
  ROOut1/1 -> Data Type Conversion/1
  Memory2/1 -> MinMax2/2
  ROOut2/1 -> Data Type Conversion1/1
  Memory1/1 -> MinMax1/2
  [out2] -> ROOut2/2
  In1/1 -> ROOut1/1
  In2/1 -> ROOut2/1
  [out1] -> ROOut1/2
  MinMax/1 -> Out1/1
  Constant3/1 -> MinMax/3

== system c00009M_harness/Eval88 ==
  In1 : Inport
  In2 : Inport  Port=2
  Constant3 : Constant
  Data Type Conversion : DataTypeConversion
  Data Type Conversion1 : DataTypeConversion
  Memory1 : Memory  InitialCondition=1
  Memory2 : Memory  InitialCondition=1
  MinMax : MinMax  Inputs=3
  MinMax1 : MinMax  Inputs=2
  MinMax2 : MinMax  Inputs=2
  ROOut1 : RelationalOperator  Operator===  OutDataTypeStr=boolean  RndMeth=Simplest
  ROOut2 : RelationalOperator  Operator===  OutDataTypeStr=boolean  RndMeth=Simplest
  Out1 : Outport
  wires:
  Data Type Conversion1/1 -> MinMax2/1
  Data Type Conversion/1 -> MinMax1/1
  MinMax1/1 -> Memory1/1, MinMax/1
  MinMax2/1 -> MinMax/2, Memory2/1
  ROOut1/1 -> Data Type Conversion/1
  Memory2/1 -> MinMax2/2
  ROOut2/1 -> Data Type Conversion1/1
  Memory1/1 -> MinMax1/2
  [out2] -> ROOut2/2
  In1/1 -> ROOut1/1
  In2/1 -> ROOut2/1
  [out1] -> ROOut1/2
  MinMax/1 -> Out1/1
  Constant3/1 -> MinMax/3

== system c00009M_harness/Eval89 ==
  In1 : Inport
  In2 : Inport  Port=2
  Constant3 : Constant
  Data Type Conversion : DataTypeConversion
  Data Type Conversion1 : DataTypeConversion
  Memory1 : Memory  InitialCondition=1
  Memory2 : Memory  InitialCondition=1
  MinMax : MinMax  Inputs=3
  MinMax1 : MinMax  Inputs=2
  MinMax2 : MinMax  Inputs=2
  ROOut1 : RelationalOperator  Operator===  OutDataTypeStr=boolean  RndMeth=Simplest
  ROOut2 : RelationalOperator  Operator===  OutDataTypeStr=boolean  RndMeth=Simplest
  Out1 : Outport
  wires:
  Data Type Conversion1/1 -> MinMax2/1
  Data Type Conversion/1 -> MinMax1/1
  MinMax1/1 -> Memory1/1, MinMax/1
  MinMax2/1 -> MinMax/2, Memory2/1
  ROOut1/1 -> Data Type Conversion/1
  Memory2/1 -> MinMax2/2
  ROOut2/1 -> Data Type Conversion1/1
  Memory1/1 -> MinMax1/2
  [out2] -> ROOut2/2
  In1/1 -> ROOut1/1
  In2/1 -> ROOut2/1
  [out1] -> ROOut1/2
  MinMax/1 -> Out1/1
  Constant3/1 -> MinMax/3

== system c00009M_harness/Eval90 ==
  In1 : Inport
  In2 : Inport  Port=2
  Constant3 : Constant
  Data Type Conversion : DataTypeConversion
  Data Type Conversion1 : DataTypeConversion
  Memory1 : Memory  InitialCondition=1
  Memory2 : Memory  InitialCondition=1
  MinMax : MinMax  Inputs=3
  MinMax1 : MinMax  Inputs=2
  MinMax2 : MinMax  Inputs=2
  ROOut1 : RelationalOperator  Operator===  OutDataTypeStr=boolean  RndMeth=Simplest
  ROOut2 : RelationalOperator  Operator===  OutDataTypeStr=boolean  RndMeth=Simplest
  Out1 : Outport
  wires:
  Data Type Conversion1/1 -> MinMax2/1
  Data Type Conversion/1 -> MinMax1/1
  MinMax1/1 -> Memory1/1, MinMax/1
  MinMax2/1 -> MinMax/2, Memory2/1
  ROOut1/1 -> Data Type Conversion/1
  Memory2/1 -> MinMax2/2
  ROOut2/1 -> Data Type Conversion1/1
  Memory1/1 -> MinMax1/2
  [out2] -> ROOut2/2
  In1/1 -> ROOut1/1
  In2/1 -> ROOut2/1
  [out1] -> ROOut1/2
  MinMax/1 -> Out1/1
  Constant3/1 -> MinMax/3

== system c00009M_harness/Eval91 ==
  In1 : Inport
  In2 : Inport  Port=2
  Constant3 : Constant
  Data Type Conversion : DataTypeConversion
  Data Type Conversion1 : DataTypeConversion
  Memory1 : Memory  InitialCondition=1
  Memory2 : Memory  InitialCondition=1
  MinMax : MinMax  Inputs=3
  MinMax1 : MinMax  Inputs=2
  MinMax2 : MinMax  Inputs=2
  ROOut1 : RelationalOperator  Operator===  OutDataTypeStr=boolean  RndMeth=Simplest
  ROOut2 : RelationalOperator  Operator===  OutDataTypeStr=boolean  RndMeth=Simplest
  Out1 : Outport
  wires:
  Data Type Conversion1/1 -> MinMax2/1
  Data Type Conversion/1 -> MinMax1/1
  MinMax1/1 -> Memory1/1, MinMax/1
  MinMax2/1 -> MinMax/2, Memory2/1
  ROOut1/1 -> Data Type Conversion/1
  Memory2/1 -> MinMax2/2
  ROOut2/1 -> Data Type Conversion1/1
  Memory1/1 -> MinMax1/2
  [out2] -> ROOut2/2
  In1/1 -> ROOut1/1
  In2/1 -> ROOut2/1
  [out1] -> ROOut1/2
  MinMax/1 -> Out1/1
  Constant3/1 -> MinMax/3

== system c00009M_harness/Eval92 ==
  In1 : Inport
  In2 : Inport  Port=2
  Constant3 : Constant
  Data Type Conversion : DataTypeConversion
  Data Type Conversion1 : DataTypeConversion
  Memory1 : Memory  InitialCondition=1
  Memory2 : Memory  InitialCondition=1
  MinMax : MinMax  Inputs=3
  MinMax1 : MinMax  Inputs=2
  MinMax2 : MinMax  Inputs=2
  ROOut1 : RelationalOperator  Operator===  OutDataTypeStr=boolean  RndMeth=Simplest
  ROOut2 : RelationalOperator  Operator===  OutDataTypeStr=boolean  RndMeth=Simplest
  Out1 : Outport
  wires:
  Data Type Conversion1/1 -> MinMax2/1
  Data Type Conversion/1 -> MinMax1/1
  MinMax1/1 -> Memory1/1, MinMax/1
  MinMax2/1 -> MinMax/2, Memory2/1
  ROOut1/1 -> Data Type Conversion/1
  Memory2/1 -> MinMax2/2
  ROOut2/1 -> Data Type Conversion1/1
  Memory1/1 -> MinMax1/2
  [out2] -> ROOut2/2
  In1/1 -> ROOut1/1
  In2/1 -> ROOut2/1
  [out1] -> ROOut1/2
  MinMax/1 -> Out1/1
  Constant3/1 -> MinMax/3

== system c00009M_harness/Eval93 ==
  In1 : Inport
  In2 : Inport  Port=2
  Constant3 : Constant
  Data Type Conversion : DataTypeConversion
  Data Type Conversion1 : DataTypeConversion
  Memory1 : Memory  InitialCondition=1
  Memory2 : Memory  InitialCondition=1
  MinMax : MinMax  Inputs=3
  MinMax1 : MinMax  Inputs=2
  MinMax2 : MinMax  Inputs=2
  ROOut1 : RelationalOperator  Operator===  OutDataTypeStr=boolean  RndMeth=Simplest
  ROOut2 : RelationalOperator  Operator===  OutDataTypeStr=boolean  RndMeth=Simplest
  Out1 : Outport
  wires:
  Data Type Conversion1/1 -> MinMax2/1
  Data Type Conversion/1 -> MinMax1/1
  MinMax1/1 -> Memory1/1, MinMax/1
  MinMax2/1 -> MinMax/2, Memory2/1
  ROOut1/1 -> Data Type Conversion/1
  Memory2/1 -> MinMax2/2
  ROOut2/1 -> Data Type Conversion1/1
  Memory1/1 -> MinMax1/2
  [out2] -> ROOut2/2
  In1/1 -> ROOut1/1
  In2/1 -> ROOut2/1
  [out1] -> ROOut1/2
  MinMax/1 -> Out1/1
  Constant3/1 -> MinMax/3

== system c00009M_harness/Eval94 ==
  In1 : Inport
  In2 : Inport  Port=2
  Constant3 : Constant
  Data Type Conversion : DataTypeConversion
  Data Type Conversion1 : DataTypeConversion
  Memory1 : Memory  InitialCondition=1
  Memory2 : Memory  InitialCondition=1
  MinMax : MinMax  Inputs=3
  MinMax1 : MinMax  Inputs=2
  MinMax2 : MinMax  Inputs=2
  ROOut1 : RelationalOperator  Operator===  OutDataTypeStr=boolean  RndMeth=Simplest
  ROOut2 : RelationalOperator  Operator===  OutDataTypeStr=boolean  RndMeth=Simplest
  Out1 : Outport
  wires:
  Data Type Conversion1/1 -> MinMax2/1
  Data Type Conversion/1 -> MinMax1/1
  MinMax1/1 -> Memory1/1, MinMax/1
  MinMax2/1 -> MinMax/2, Memory2/1
  ROOut1/1 -> Data Type Conversion/1
  Memory2/1 -> MinMax2/2
  ROOut2/1 -> Data Type Conversion1/1
  Memory1/1 -> MinMax1/2
  [out2] -> ROOut2/2
  In1/1 -> ROOut1/1
  In2/1 -> ROOut2/1
  [out1] -> ROOut1/2
  MinMax/1 -> Out1/1
  Constant3/1 -> MinMax/3

== system c00009M_harness/Eval95 ==
  In1 : Inport
  In2 : Inport  Port=2
  Constant3 : Constant
  Data Type Conversion : DataTypeConversion
  Data Type Conversion1 : DataTypeConversion
  Memory1 : Memory  InitialCondition=1
  Memory2 : Memory  InitialCondition=1
  MinMax : MinMax  Inputs=3
  MinMax1 : MinMax  Inputs=2
  MinMax2 : MinMax  Inputs=2
  ROOut1 : RelationalOperator  Operator===  OutDataTypeStr=boolean  RndMeth=Simplest
  ROOut2 : RelationalOperator  Operator===  OutDataTypeStr=boolean  RndMeth=Simplest
  Out1 : Outport
  wires:
  Data Type Conversion1/1 -> MinMax2/1
  Data Type Conversion/1 -> MinMax1/1
  MinMax1/1 -> Memory1/1, MinMax/1
  MinMax2/1 -> MinMax/2, Memory2/1
  ROOut1/1 -> Data Type Conversion/1
  Memory2/1 -> MinMax2/2
  ROOut2/1 -> Data Type Conversion1/1
  Memory1/1 -> MinMax1/2
  [out2] -> ROOut2/2
  In1/1 -> ROOut1/1
  In2/1 -> ROOut2/1
  [out1] -> ROOut1/2
  MinMax/1 -> Out1/1
  Constant3/1 -> MinMax/3

== system c00009M_harness/Eval96 ==
  In1 : Inport
  In2 : Inport  Port=2
  Constant3 : Constant
  Data Type Conversion : DataTypeConversion
  Data Type Conversion1 : DataTypeConversion
  Memory1 : Memory  InitialCondition=1
  Memory2 : Memory  InitialCondition=1
  MinMax : MinMax  Inputs=3
  MinMax1 : MinMax  Inputs=2
  MinMax2 : MinMax  Inputs=2
  ROOut1 : RelationalOperator  Operator===  OutDataTypeStr=boolean  RndMeth=Simplest
  ROOut2 : RelationalOperator  Operator===  OutDataTypeStr=boolean  RndMeth=Simplest
  Out1 : Outport
  wires:
  Data Type Conversion1/1 -> MinMax2/1
  Data Type Conversion/1 -> MinMax1/1
  MinMax1/1 -> Memory1/1, MinMax/1
  MinMax2/1 -> MinMax/2, Memory2/1
  ROOut1/1 -> Data Type Conversion/1
  Memory2/1 -> MinMax2/2
  ROOut2/1 -> Data Type Conversion1/1
  Memory1/1 -> MinMax1/2
  [out2] -> ROOut2/2
  In1/1 -> ROOut1/1
  In2/1 -> ROOut2/1
  [out1] -> ROOut1/2
  MinMax/1 -> Out1/1
  Constant3/1 -> MinMax/3
